simulink model "Model_InterpretationEngine64"  (R2022b)
settings: Solver=FixedStepDiscrete  StartTime=0.0  StopTime=5  RelTol=1e-3  EnableMultiTasking=on
InitFcn:
  | % Initialize model
  | ModelSettings=BTConfig.GetModelSettings();
  | 
  | ModelSettings.Validate();
  | 
  | ModelInit;
  | 
  | 
  | % load library data
  | GainLibrary_data;
  | % Load saved values from partition process
  | CapturedConstMask.LoadMapFromFile(bdroot)
  | % Load saved values from partition process
  | TSP_Mask.LoadMapFromFile(bdroot)
StartFcn:
  | % make sure all the simulated RTC requests are found
  | %RTC_SIM_OBJ.ValidateREQs();
undefined symbols (not defined in the file or in its folder): NumHFRefBPF, NumHFRefLPF
libraries: StateVar x112, TSP x56, FeaturePath x24
(part 2 of 5)

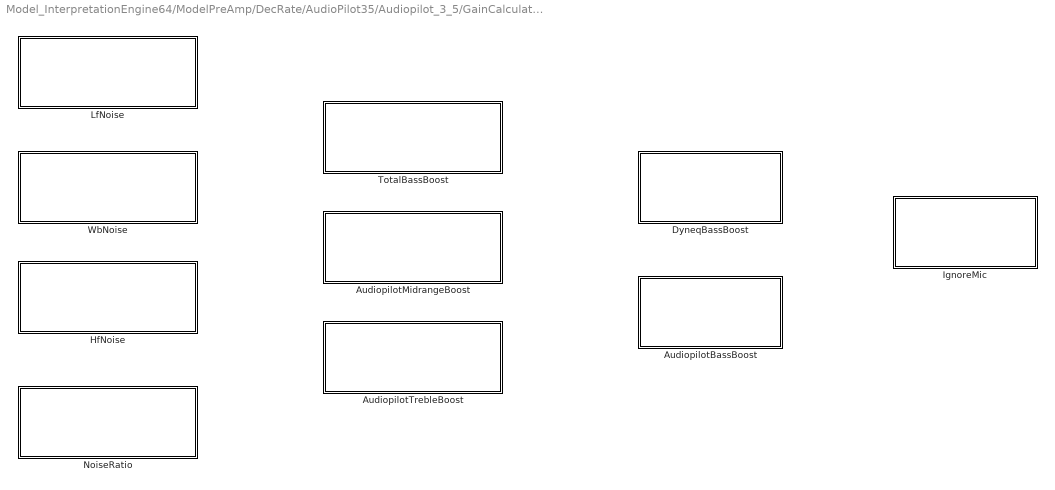
== system Model_InterpretationEngine64/ModelPreAmp/DecRate/AudioPilot35/Audiopilot_3_5/GainCalculation/Monitoring ==
  AudiopilotBassBoost : Subsystem  mask(Talaria Target State Variable){TriggerInit=[375 166 515 234], TspName=AudiopilotBassBoostDb, StateName=AudiopilotBassBoostDb, UseSameName=on, IfdefMacro=[]}
      mask prompts: TriggerInit "Hidden: MoveFcn redraw"; TspName "Name:"; StateName "Name of StateVar:"; UseSameName "Use same name for state variable and TSP"; IfdefMacro "Additional #ifdef macro to enable trigger capture:"
      mask help: The TargetStateVar block encapsultes a Target State Probe (TSP), a State Variable, and a Trivial Interpretation between them.
      mask init:
      | [ok,tspPath,activeStatePath] = TargetStateVarMask.Init(gcbh);
      settings: MoveFcn=TargetStateVarMask.CB_TriggerInit(gcbh);
      mask Help: See help for StateVar and TSP blocks
      mask Callback TriggerInit: TargetStateVarMask.CB_TriggerInit(gcbh);
      mask TypeOptions TspName: TSP/TspName
      mask TypeOptions StateName: StateVar/StateName
      mask Callback UseSameName: TargetStateVarMask.CB_UseSameName(gcbh);
      mask TypeOptions IfdefMacro: TSP/IfdefMacro
      mask DialogControl AdvancedPanel Prompt: Advanced
      mask DialogControl ConvertToFullInterpretation Prompt: Irreversible conversion to full interpretation
      mask DialogControl ConvertToFullInterpretation Callback: TargetStateVarMask.CB_ConvertToFullInterpretation(gcbh);
      mask DialogControl ErrorContainer Prompt: Error Messages
      mask DialogControl ErrorText Prompt: The interpreted StateVar value is not yet available
      mask DialogControl TspPathText Prompt: TSP: Current parameter name: [AudiopilotAudiopilotBassBoostDb]
      mask Display:
      | % retrieve icon definition
      | [path,w,h] = TargetStateVarMask.Icon();
      | 
      | % retrieve the block's pixel size
      | pos = get(gcbh,'position');
      | bw = pos(3) - pos(1);
      | bh = pos(4) - pos(2);
      | 
      | % draw centered icon
      | xAdj = bw/2 - w/2 + 5;
      | yAdj = bh/2 - h/2 + 4;
      | for i=1:length(path)
      | 	patch(path(i).x+xAdj, path(i).y+yAdj, path(i).rgb);
      | end
      | 
      | % show the top name or an X
      | if (exist('ok','var') && ok)
      | 	text(bw*0.5, bh*0.2, tspPath, 'horizontalAlignment', 'center');
      | 	patch(0,0,[1 1 1]);
      | 	patch(bw,bh,[1 1 1]);
      | else
      | 	tx=bw*0.03;
      | 	ty=bh*0.03;
      | 	patch([0 tx bw bw-tx], [ty 0 bh-ty bh], [1 0 0]);
      | 	patch([0 bw-tx bw tx], [bh-ty 0 ty bh], [1 0 0]);
      | end
  AudiopilotMidrangeBoost : Subsystem  mask(Talaria Target State Variable){TriggerInit=[60 101 235 169], TspName=AudiopilotMidrangeBoostDb, StateName=AudiopilotMidrangeBoostDb, UseSameName=on, IfdefMacro=[]}
      mask prompts: TriggerInit "Hidden: MoveFcn redraw"; TspName "Name:"; StateName "Name of StateVar:"; UseSameName "Use same name for state variable and TSP"; IfdefMacro "Additional #ifdef macro to enable trigger capture:"
      mask help: The TargetStateVar block encapsultes a Target State Probe (TSP), a State Variable, and a Trivial Interpretation between them.
      mask init:
      | [ok,tspPath,activeStatePath] = TargetStateVarMask.Init(gcbh);
      settings: MoveFcn=TargetStateVarMask.CB_TriggerInit(gcbh);
      mask Help: See help for StateVar and TSP blocks
      mask Callback TriggerInit: TargetStateVarMask.CB_TriggerInit(gcbh);
      mask TypeOptions TspName: TSP/TspName
      mask TypeOptions StateName: StateVar/StateName
      mask Callback UseSameName: TargetStateVarMask.CB_UseSameName(gcbh);
      mask TypeOptions IfdefMacro: TSP/IfdefMacro
      mask DialogControl AdvancedPanel Prompt: Advanced
      mask DialogControl ConvertToFullInterpretation Prompt: Irreversible conversion to full interpretation
      mask DialogControl ConvertToFullInterpretation Callback: TargetStateVarMask.CB_ConvertToFullInterpretation(gcbh);
      mask DialogControl ErrorContainer Prompt: Error Messages
      mask DialogControl ErrorText Prompt: The interpreted StateVar value is not yet available
      mask DialogControl TspPathText Prompt: TSP: Current parameter name: [AudiopilotAudiopilotMidrangeBoostDb]
      mask Display:
      | % retrieve icon definition
      | [path,w,h] = TargetStateVarMask.Icon();
      | 
      | % retrieve the block's pixel size
      | pos = get(gcbh,'position');
      | bw = pos(3) - pos(1);
      | bh = pos(4) - pos(2);
      | 
      | % draw centered icon
      | xAdj = bw/2 - w/2 + 5;
      | yAdj = bh/2 - h/2 + 4;
      | for i=1:length(path)
      | 	patch(path(i).x+xAdj, path(i).y+yAdj, path(i).rgb);
      | end
      | 
      | % show the top name or an X
      | if (exist('ok','var') && ok)
      | 	text(bw*0.5, bh*0.2, tspPath, 'horizontalAlignment', 'center');
      | 	patch(0,0,[1 1 1]);
      | 	patch(bw,bh,[1 1 1]);
      | else
      | 	tx=bw*0.03;
      | 	ty=bh*0.03;
      | 	patch([0 tx bw bw-tx], [ty 0 bh-ty bh], [1 0 0]);
      | 	patch([0 bw-tx bw tx], [bh-ty 0 ty bh], [1 0 0]);
      | end
  AudiopilotTrebleBoost : Subsystem  mask(Talaria Target State Variable){TriggerInit=[60 211 235 279], TspName=AudiopilotTrebleBoostDb, StateName=AudiopilotTrebleBoostDb, UseSameName=on, IfdefMacro=[]}
      mask prompts: TriggerInit "Hidden: MoveFcn redraw"; TspName "Name:"; StateName "Name of StateVar:"; UseSameName "Use same name for state variable and TSP"; IfdefMacro "Additional #ifdef macro to enable trigger capture:"
      mask help: The TargetStateVar block encapsultes a Target State Probe (TSP), a State Variable, and a Trivial Interpretation between them.
      mask init:
      | [ok,tspPath,activeStatePath] = TargetStateVarMask.Init(gcbh);
      settings: MoveFcn=TargetStateVarMask.CB_TriggerInit(gcbh);
      mask Help: See help for StateVar and TSP blocks
      mask Callback TriggerInit: TargetStateVarMask.CB_TriggerInit(gcbh);
      mask TypeOptions TspName: TSP/TspName
      mask TypeOptions StateName: StateVar/StateName
      mask Callback UseSameName: TargetStateVarMask.CB_UseSameName(gcbh);
      mask TypeOptions IfdefMacro: TSP/IfdefMacro
      mask DialogControl AdvancedPanel Prompt: Advanced
      mask DialogControl ConvertToFullInterpretation Prompt: Irreversible conversion to full interpretation
      mask DialogControl ConvertToFullInterpretation Callback: TargetStateVarMask.CB_ConvertToFullInterpretation(gcbh);
      mask DialogControl ErrorContainer Prompt: Error Messages
      mask DialogControl ErrorText Prompt: The interpreted StateVar value is not yet available
      mask DialogControl TspPathText Prompt: TSP: Current parameter name: [AudiopilotAudiopilotTrebleBoostDb]
      mask Display:
      | % retrieve icon definition
      | [path,w,h] = TargetStateVarMask.Icon();
      | 
      | % retrieve the block's pixel size
      | pos = get(gcbh,'position');
      | bw = pos(3) - pos(1);
      | bh = pos(4) - pos(2);
      | 
      | % draw centered icon
      | xAdj = bw/2 - w/2 + 5;
      | yAdj = bh/2 - h/2 + 4;
      | for i=1:length(path)
      | 	patch(path(i).x+xAdj, path(i).y+yAdj, path(i).rgb);
      | end
      | 
      | % show the top name or an X
      | if (exist('ok','var') && ok)
      | 	text(bw*0.5, bh*0.2, tspPath, 'horizontalAlignment', 'center');
      | 	patch(0,0,[1 1 1]);
      | 	patch(bw,bh,[1 1 1]);
      | else
      | 	tx=bw*0.03;
      | 	ty=bh*0.03;
      | 	patch([0 tx bw bw-tx], [ty 0 bh-ty bh], [1 0 0]);
      | 	patch([0 bw-tx bw tx], [bh-ty 0 ty bh], [1 0 0]);
      | end
  DyneqBassBoost : Subsystem  mask(Talaria Target State Variable){TriggerInit=[375 41 515 109], TspName=DyneqBassBoostDb, StateName=DyneqBassBoostDb, UseSameName=on, IfdefMacro=[]}
      mask prompts: TriggerInit "Hidden: MoveFcn redraw"; TspName "Name:"; StateName "Name of StateVar:"; UseSameName "Use same name for state variable and TSP"; IfdefMacro "Additional #ifdef macro to enable trigger capture:"
      mask help: The TargetStateVar block encapsultes a Target State Probe (TSP), a State Variable, and a Trivial Interpretation between them.
      mask init:
      | [ok,tspPath,activeStatePath] = TargetStateVarMask.Init(gcbh);
      settings: MoveFcn=TargetStateVarMask.CB_TriggerInit(gcbh);
      mask Help: See help for StateVar and TSP blocks
      mask Callback TriggerInit: TargetStateVarMask.CB_TriggerInit(gcbh);
      mask TypeOptions TspName: TSP/TspName
      mask TypeOptions StateName: StateVar/StateName
      mask Callback UseSameName: TargetStateVarMask.CB_UseSameName(gcbh);
      mask TypeOptions IfdefMacro: TSP/IfdefMacro
      mask DialogControl AdvancedPanel Prompt: Advanced
      mask DialogControl ConvertToFullInterpretation Prompt: Irreversible conversion to full interpretation
      mask DialogControl ConvertToFullInterpretation Callback: TargetStateVarMask.CB_ConvertToFullInterpretation(gcbh);
      mask DialogControl ErrorContainer Prompt: Error Messages
      mask DialogControl ErrorText Prompt: The interpreted StateVar value is not yet available
      mask DialogControl TspPathText Prompt: TSP: Current parameter name: [AudiopilotDyneqBassBoostDb]
      mask Display:
      | % retrieve icon definition
      | [path,w,h] = TargetStateVarMask.Icon();
      | 
      | % retrieve the block's pixel size
      | pos = get(gcbh,'position');
      | bw = pos(3) - pos(1);
      | bh = pos(4) - pos(2);
      | 
      | % draw centered icon
      | xAdj = bw/2 - w/2 + 5;
      | yAdj = bh/2 - h/2 + 4;
      | for i=1:length(path)
      | 	patch(path(i).x+xAdj, path(i).y+yAdj, path(i).rgb);
      | end
      | 
      | % show the top name or an X
      | if (exist('ok','var') && ok)
      | 	text(bw*0.5, bh*0.2, tspPath, 'horizontalAlignment', 'center');
      | 	patch(0,0,[1 1 1]);
      | 	patch(bw,bh,[1 1 1]);
      | else
      | 	tx=bw*0.03;
      | 	ty=bh*0.03;
      | 	patch([0 tx bw bw-tx], [ty 0 bh-ty bh], [1 0 0]);
      | 	patch([0 bw-tx bw tx], [bh-ty 0 ty bh], [1 0 0]);
      | end
  HfNoise : Subsystem  mask(Talaria Target State Variable){TriggerInit=[-245 151 -70 219], TspName=HfNoiseDbspl, StateName=HfNoiseDbspl, UseSameName=on, IfdefMacro=[]}
      mask prompts: TriggerInit "Hidden: MoveFcn redraw"; TspName "Name:"; StateName "Name of StateVar:"; UseSameName "Use same name for state variable and TSP"; IfdefMacro "Additional #ifdef macro to enable trigger capture:"
      mask help: The TargetStateVar block encapsultes a Target State Probe (TSP), a State Variable, and a Trivial Interpretation between them.
      mask init:
      | [ok,tspPath,activeStatePath] = TargetStateVarMask.Init(gcbh);
      settings: MoveFcn=TargetStateVarMask.CB_TriggerInit(gcbh);
      mask Help: See help for StateVar and TSP blocks
      mask Callback TriggerInit: TargetStateVarMask.CB_TriggerInit(gcbh);
      mask TypeOptions TspName: TSP/TspName
      mask TypeOptions StateName: StateVar/StateName
      mask Callback UseSameName: TargetStateVarMask.CB_UseSameName(gcbh);
      mask TypeOptions IfdefMacro: TSP/IfdefMacro
      mask DialogControl AdvancedPanel Prompt: Advanced
      mask DialogControl ConvertToFullInterpretation Prompt: Irreversible conversion to full interpretation
      mask DialogControl ConvertToFullInterpretation Callback: TargetStateVarMask.CB_ConvertToFullInterpretation(gcbh);
      mask DialogControl ErrorContainer Prompt: Error Messages
      mask DialogControl ErrorText Prompt: The interpreted StateVar value is not yet available
      mask DialogControl TspPathText Prompt: TSP: Current parameter name: [AudiopilotHfNoiseDbspl]
      mask Display:
      | % retrieve icon definition
      | [path,w,h] = TargetStateVarMask.Icon();
      | 
      | % retrieve the block's pixel size
      | pos = get(gcbh,'position');
      | bw = pos(3) - pos(1);
      | bh = pos(4) - pos(2);
      | 
      | % draw centered icon
      | xAdj = bw/2 - w/2 + 5;
      | yAdj = bh/2 - h/2 + 4;
      | for i=1:length(path)
      | 	patch(path(i).x+xAdj, path(i).y+yAdj, path(i).rgb);
      | end
      | 
      | % show the top name or an X
      | if (exist('ok','var') && ok)
      | 	text(bw*0.5, bh*0.2, tspPath, 'horizontalAlignment', 'center');
      | 	patch(0,0,[1 1 1]);
      | 	patch(bw,bh,[1 1 1]);
      | else
      | 	tx=bw*0.03;
      | 	ty=bh*0.03;
      | 	patch([0 tx bw bw-tx], [ty 0 bh-ty bh], [1 0 0]);
      | 	patch([0 bw-tx bw tx], [bh-ty 0 ty bh], [1 0 0]);
      | end
  IgnoreMic : Subsystem  mask(Talaria Target State Variable){TriggerInit=[630 86 770 154], TspName=IgnoreMicFlag, StateName=IgnoreMicFlag, UseSameName=on, IfdefMacro=[]}
      mask prompts: TriggerInit "Hidden: MoveFcn redraw"; TspName "Name:"; StateName "Name of StateVar:"; UseSameName "Use same name for state variable and TSP"; IfdefMacro "Additional #ifdef macro to enable trigger capture:"
      mask help: The TargetStateVar block encapsultes a Target State Probe (TSP), a State Variable, and a Trivial Interpretation between them.
      mask init:
      | [ok,tspPath,activeStatePath] = TargetStateVarMask.Init(gcbh);
      settings: MoveFcn=TargetStateVarMask.CB_TriggerInit(gcbh);
      mask Help: See help for StateVar and TSP blocks
      mask Callback TriggerInit: TargetStateVarMask.CB_TriggerInit(gcbh);
      mask TypeOptions TspName: TSP/TspName
      mask TypeOptions StateName: StateVar/StateName
      mask Callback UseSameName: TargetStateVarMask.CB_UseSameName(gcbh);
      mask TypeOptions IfdefMacro: TSP/IfdefMacro
      mask DialogControl AdvancedPanel Prompt: Advanced
      mask DialogControl ConvertToFullInterpretation Prompt: Irreversible conversion to full interpretation
      mask DialogControl ConvertToFullInterpretation Callback: TargetStateVarMask.CB_ConvertToFullInterpretation(gcbh);
      mask DialogControl ErrorContainer Prompt: Error Messages
      mask DialogControl ErrorText Prompt: The interpreted StateVar value is not yet available
      mask DialogControl TspPathText Prompt: TSP: Current parameter name: [AudiopilotIgnoreMicFlag]
      mask Display:
      | % retrieve icon definition
      | [path,w,h] = TargetStateVarMask.Icon();
      | 
      | % retrieve the block's pixel size
      | pos = get(gcbh,'position');
      | bw = pos(3) - pos(1);
      | bh = pos(4) - pos(2);
      | 
      | % draw centered icon
      | xAdj = bw/2 - w/2 + 5;
      | yAdj = bh/2 - h/2 + 4;
      | for i=1:length(path)
      | 	patch(path(i).x+xAdj, path(i).y+yAdj, path(i).rgb);
      | end
      | 
      | % show the top name or an X
      | if (exist('ok','var') && ok)
      | 	text(bw*0.5, bh*0.2, tspPath, 'horizontalAlignment', 'center');
      | 	patch(0,0,[1 1 1]);
      | 	patch(bw,bh,[1 1 1]);
      | else
      | 	tx=bw*0.03;
      | 	ty=bh*0.03;
      | 	patch([0 tx bw bw-tx], [ty 0 bh-ty bh], [1 0 0]);
      | 	patch([0 bw-tx bw tx], [bh-ty 0 ty bh], [1 0 0]);
      | end
  LfNoise : Subsystem  mask(Talaria Target State Variable){TriggerInit=[-245 -74 -70 -6], TspName=LfNoiseDbspl, StateName=LfNoiseDbspl, UseSameName=on, IfdefMacro=[]}
      mask prompts: TriggerInit "Hidden: MoveFcn redraw"; TspName "Name:"; StateName "Name of StateVar:"; UseSameName "Use same name for state variable and TSP"; IfdefMacro "Additional #ifdef macro to enable trigger capture:"
      mask help: The TargetStateVar block encapsultes a Target State Probe (TSP), a State Variable, and a Trivial Interpretation between them.
      mask init:
      | [ok,tspPath,activeStatePath] = TargetStateVarMask.Init(gcbh);
      settings: MoveFcn=TargetStateVarMask.CB_TriggerInit(gcbh);
      mask Help: See help for StateVar and TSP blocks
      mask Callback TriggerInit: TargetStateVarMask.CB_TriggerInit(gcbh);
      mask TypeOptions TspName: TSP/TspName
      mask TypeOptions StateName: StateVar/StateName
      mask Callback UseSameName: TargetStateVarMask.CB_UseSameName(gcbh);
      mask TypeOptions IfdefMacro: TSP/IfdefMacro
      mask DialogControl AdvancedPanel Prompt: Advanced
      mask DialogControl ConvertToFullInterpretation Prompt: Irreversible conversion to full interpretation
      mask DialogControl ConvertToFullInterpretation Callback: TargetStateVarMask.CB_ConvertToFullInterpretation(gcbh);
      mask DialogControl ErrorContainer Prompt: Error Messages
      mask DialogControl ErrorText Prompt: The interpreted StateVar value is not yet available
      mask DialogControl TspPathText Prompt: TSP: Current parameter name: [AudiopilotLfNoiseDbspl]
      mask Display:
      | % retrieve icon definition
      | [path,w,h] = TargetStateVarMask.Icon();
      | 
      | % retrieve the block's pixel size
      | pos = get(gcbh,'position');
      | bw = pos(3) - pos(1);
      | bh = pos(4) - pos(2);
      | 
      | % draw centered icon
      | xAdj = bw/2 - w/2 + 5;
      | yAdj = bh/2 - h/2 + 4;
      | for i=1:length(path)
      | 	patch(path(i).x+xAdj, path(i).y+yAdj, path(i).rgb);
      | end
      | 
      | % show the top name or an X
      | if (exist('ok','var') && ok)
      | 	text(bw*0.5, bh*0.2, tspPath, 'horizontalAlignment', 'center');
      | 	patch(0,0,[1 1 1]);
      | 	patch(bw,bh,[1 1 1]);
      | else
      | 	tx=bw*0.03;
      | 	ty=bh*0.03;
      | 	patch([0 tx bw bw-tx], [ty 0 bh-ty bh], [1 0 0]);
      | 	patch([0 bw-tx bw tx], [bh-ty 0 ty bh], [1 0 0]);
      | end
  NoiseRatio : Subsystem  mask(Talaria Target State Variable){TriggerInit=[-245 276 -70 344], TspName=NoiseRatio, StateName=NoiseRatio, UseSameName=on, IfdefMacro=[]}
      mask prompts: TriggerInit "Hidden: MoveFcn redraw"; TspName "Name:"; StateName "Name of StateVar:"; UseSameName "Use same name for state variable and TSP"; IfdefMacro "Additional #ifdef macro to enable trigger capture:"
      mask help: The TargetStateVar block encapsultes a Target State Probe (TSP), a State Variable, and a Trivial Interpretation between them.
      mask init:
      | [ok,tspPath,activeStatePath] = TargetStateVarMask.Init(gcbh);
      settings: MoveFcn=TargetStateVarMask.CB_TriggerInit(gcbh);
      mask Help: See help for StateVar and TSP blocks
      mask Callback TriggerInit: TargetStateVarMask.CB_TriggerInit(gcbh);
      mask TypeOptions TspName: TSP/TspName
      mask TypeOptions StateName: StateVar/StateName
      mask Callback UseSameName: TargetStateVarMask.CB_UseSameName(gcbh);
      mask TypeOptions IfdefMacro: TSP/IfdefMacro
      mask DialogControl AdvancedPanel Prompt: Advanced
      mask DialogControl ConvertToFullInterpretation Prompt: Irreversible conversion to full interpretation
      mask DialogControl ConvertToFullInterpretation Callback: TargetStateVarMask.CB_ConvertToFullInterpretation(gcbh);
      mask DialogControl ErrorContainer Prompt: Error Messages
      mask DialogControl ErrorText Prompt: The interpreted StateVar value is not yet available
      mask DialogControl TspPathText Prompt: TSP: Current parameter name: [AudiopilotNoiseRatio]
      mask Display:
      | % retrieve icon definition
      | [path,w,h] = TargetStateVarMask.Icon();
      | 
      | % retrieve the block's pixel size
      | pos = get(gcbh,'position');
      | bw = pos(3) - pos(1);
      | bh = pos(4) - pos(2);
      | 
      | % draw centered icon
      | xAdj = bw/2 - w/2 + 5;
      | yAdj = bh/2 - h/2 + 4;
      | for i=1:length(path)
      | 	patch(path(i).x+xAdj, path(i).y+yAdj, path(i).rgb);
      | end
      | 
      | % show the top name or an X
      | if (exist('ok','var') && ok)
      | 	text(bw*0.5, bh*0.2, tspPath, 'horizontalAlignment', 'center');
      | 	patch(0,0,[1 1 1]);
      | 	patch(bw,bh,[1 1 1]);
      | else
      | 	tx=bw*0.03;
      | 	ty=bh*0.03;
      | 	patch([0 tx bw bw-tx], [ty 0 bh-ty bh], [1 0 0]);
      | 	patch([0 bw-tx bw tx], [bh-ty 0 ty bh], [1 0 0]);
      | end
  TotalBassBoost : Subsystem  mask(Talaria Target State Variable){TriggerInit=[60 -9 235 59], TspName=TotalBassBoostDb, StateName=TotalBassBoostDb, UseSameName=on, IfdefMacro=[]}
      mask prompts: TriggerInit "Hidden: MoveFcn redraw"; TspName "Name:"; StateName "Name of StateVar:"; UseSameName "Use same name for state variable and TSP"; IfdefMacro "Additional #ifdef macro to enable trigger capture:"
      mask help: The TargetStateVar block encapsultes a Target State Probe (TSP), a State Variable, and a Trivial Interpretation between them.
      mask init:
      | [ok,tspPath,activeStatePath] = TargetStateVarMask.Init(gcbh);
      settings: MoveFcn=TargetStateVarMask.CB_TriggerInit(gcbh);
      mask Help: See help for StateVar and TSP blocks
      mask Callback TriggerInit: TargetStateVarMask.CB_TriggerInit(gcbh);
      mask TypeOptions TspName: TSP/TspName
      mask TypeOptions StateName: StateVar/StateName
      mask Callback UseSameName: TargetStateVarMask.CB_UseSameName(gcbh);
      mask TypeOptions IfdefMacro: TSP/IfdefMacro
      mask DialogControl AdvancedPanel Prompt: Advanced
      mask DialogControl ConvertToFullInterpretation Prompt: Irreversible conversion to full interpretation
      mask DialogControl ConvertToFullInterpretation Callback: TargetStateVarMask.CB_ConvertToFullInterpretation(gcbh);
      mask DialogControl ErrorContainer Prompt: Error Messages
      mask DialogControl ErrorText Prompt: The interpreted StateVar value is not yet available
      mask DialogControl TspPathText Prompt: TSP: Current parameter name: [AudiopilotTotalBassBoostDb]
      mask Display:
      | % retrieve icon definition
      | [path,w,h] = TargetStateVarMask.Icon();
      | 
      | % retrieve the block's pixel size
      | pos = get(gcbh,'position');
      | bw = pos(3) - pos(1);
      | bh = pos(4) - pos(2);
      | 
      | % draw centered icon
      | xAdj = bw/2 - w/2 + 5;
      | yAdj = bh/2 - h/2 + 4;
      | for i=1:length(path)
      | 	patch(path(i).x+xAdj, path(i).y+yAdj, path(i).rgb);
      | end
      | 
      | % show the top name or an X
      | if (exist('ok','var') && ok)
      | 	text(bw*0.5, bh*0.2, tspPath, 'horizontalAlignment', 'center');
      | 	patch(0,0,[1 1 1]);
      | 	patch(bw,bh,[1 1 1]);
      | else
      | 	tx=bw*0.03;
      | 	ty=bh*0.03;
      | 	patch([0 tx bw bw-tx], [ty 0 bh-ty bh], [1 0 0]);
      | 	patch([0 bw-tx bw tx], [bh-ty 0 ty bh], [1 0 0]);
      | end
  WbNoise : Subsystem  mask(Talaria Target State Variable){TriggerInit=[-245 41 -70 109], TspName=WbNoiseDbspl, StateName=WbNoiseDbspl, UseSameName=on, IfdefMacro=[]}
      mask prompts: TriggerInit "Hidden: MoveFcn redraw"; TspName "Name:"; StateName "Name of StateVar:"; UseSameName "Use same name for state variable and TSP"; IfdefMacro "Additional #ifdef macro to enable trigger capture:"
      mask help: The TargetStateVar block encapsultes a Target State Probe (TSP), a State Variable, and a Trivial Interpretation between them.
      mask init:
      | [ok,tspPath,activeStatePath] = TargetStateVarMask.Init(gcbh);
      settings: MoveFcn=TargetStateVarMask.CB_TriggerInit(gcbh);
      mask Help: See help for StateVar and TSP blocks
      mask Callback TriggerInit: TargetStateVarMask.CB_TriggerInit(gcbh);
      mask TypeOptions TspName: TSP/TspName
      mask TypeOptions StateName: StateVar/StateName
      mask Callback UseSameName: TargetStateVarMask.CB_UseSameName(gcbh);
      mask TypeOptions IfdefMacro: TSP/IfdefMacro
      mask DialogControl AdvancedPanel Prompt: Advanced
      mask DialogControl ConvertToFullInterpretation Prompt: Irreversible conversion to full interpretation
      mask DialogControl ConvertToFullInterpretation Callback: TargetStateVarMask.CB_ConvertToFullInterpretation(gcbh);
      mask DialogControl ErrorContainer Prompt: Error Messages
      mask DialogControl ErrorText Prompt: The interpreted StateVar value is not yet available
      mask DialogControl TspPathText Prompt: TSP: Current parameter name: [AudiopilotWbNoiseDbspl]
      mask Display:
      | % retrieve icon definition
      | [path,w,h] = TargetStateVarMask.Icon();
      | 
      | % retrieve the block's pixel size
      | pos = get(gcbh,'position');
      | bw = pos(3) - pos(1);
      | bh = pos(4) - pos(2);
      | 
      | % draw centered icon
      | xAdj = bw/2 - w/2 + 5;
      | yAdj = bh/2 - h/2 + 4;
      | for i=1:length(path)
      | 	patch(path(i).x+xAdj, path(i).y+yAdj, path(i).rgb);
      | end
      | 
      | % show the top name or an X
      | if (exist('ok','var') && ok)
      | 	text(bw*0.5, bh*0.2, tspPath, 'horizontalAlignment', 'center');
      | 	patch(0,0,[1 1 1]);
      | 	patch(bw,bh,[1 1 1]);
      | else
      | 	tx=bw*0.03;
      | 	ty=bh*0.03;
      | 	patch([0 tx bw bw-tx], [ty 0 bh-ty bh], [1 0 0]);
      | 	patch([0 bw-tx bw tx], [bh-ty 0 ty bh], [1 0 0]);
      | end

== system Model_InterpretationEngine64/ModelPreAmp/DecRate/AudioPilot35/Audiopilot_3_5/GainCalculation/RampedEnable ==
  audiopilot boost gain : Subsystem  mask(Talaria Target State Variable){TriggerInit=[185 -359 325 -291], TspName=AudiopilotBoostGain, StateName=AudiopilotBoostGain, UseSameName=on, IfdefMacro=[]}
      mask prompts: TriggerInit "Hidden: MoveFcn redraw"; TspName "Name:"; StateName "Name of StateVar:"; UseSameName "Use same name for state variable and TSP"; IfdefMacro "Additional #ifdef macro to enable trigger capture:"
      mask help: The TargetStateVar block encapsultes a Target State Probe (TSP), a State Variable, and a Trivial Interpretation between them.
      mask init:
      | [ok,tspPath,activeStatePath] = TargetStateVarMask.Init(gcbh);
      settings: MoveFcn=TargetStateVarMask.CB_TriggerInit(gcbh);
      mask Help: See help for StateVar and TSP blocks
      mask Callback TriggerInit: TargetStateVarMask.CB_TriggerInit(gcbh);
      mask TypeOptions TspName: TSP/TspName
      mask TypeOptions StateName: StateVar/StateName
      mask Callback UseSameName: TargetStateVarMask.CB_UseSameName(gcbh);
      mask TypeOptions IfdefMacro: TSP/IfdefMacro
      mask DialogControl AdvancedPanel Prompt: Advanced
      mask DialogControl ConvertToFullInterpretation Prompt: Irreversible conversion to full interpretation
      mask DialogControl ConvertToFullInterpretation Callback: TargetStateVarMask.CB_ConvertToFullInterpretation(gcbh);
      mask DialogControl ErrorContainer Prompt: Error Messages
      mask DialogControl ErrorText Prompt: The interpreted StateVar value is not yet available
      mask DialogControl TspPathText Prompt: TSP: Current parameter name: [AudiopilotAudiopilotBoostGain]
      mask Display:
      | % retrieve icon definition
      | [path,w,h] = TargetStateVarMask.Icon();
      | 
      | % retrieve the block's pixel size
      | pos = get(gcbh,'position');
      | bw = pos(3) - pos(1);
      | bh = pos(4) - pos(2);
      | 
      | % draw centered icon
      | xAdj = bw/2 - w/2 + 5;
      | yAdj = bh/2 - h/2 + 4;
      | for i=1:length(path)
      | 	patch(path(i).x+xAdj, path(i).y+yAdj, path(i).rgb);
      | end
      | 
      | % show the top name or an X
      | if (exist('ok','var') && ok)
      | 	text(bw*0.5, bh*0.2, tspPath, 'horizontalAlignment', 'center');
      | 	patch(0,0,[1 1 1]);
      | 	patch(bw,bh,[1 1 1]);
      | else
      | 	tx=bw*0.03;
      | 	ty=bh*0.03;
      | 	patch([0 tx bw bw-tx], [ty 0 bh-ty bh], [1 0 0]);
      | 	patch([0 bw-tx bw tx], [bh-ty 0 ty bh], [1 0 0]);
      | end
  dyneq boost gain : Subsystem  mask(Talaria Target State Variable){TriggerInit=[185 -454 325 -386], TspName=DyneqBoostGain, StateName=DyneqBoostGain, UseSameName=on, IfdefMacro=[]}
      mask prompts: TriggerInit "Hidden: MoveFcn redraw"; TspName "Name:"; StateName "Name of StateVar:"; UseSameName "Use same name for state variable and TSP"; IfdefMacro "Additional #ifdef macro to enable trigger capture:"
      mask help: The TargetStateVar block encapsultes a Target State Probe (TSP), a State Variable, and a Trivial Interpretation between them.
      mask init:
      | [ok,tspPath,activeStatePath] = TargetStateVarMask.Init(gcbh);
      settings: MoveFcn=TargetStateVarMask.CB_TriggerInit(gcbh);
      mask Help: See help for StateVar and TSP blocks
      mask Callback TriggerInit: TargetStateVarMask.CB_TriggerInit(gcbh);
      mask TypeOptions TspName: TSP/TspName
      mask TypeOptions StateName: StateVar/StateName
      mask Callback UseSameName: TargetStateVarMask.CB_UseSameName(gcbh);
      mask TypeOptions IfdefMacro: TSP/IfdefMacro
      mask DialogControl AdvancedPanel Prompt: Advanced
      mask DialogControl ConvertToFullInterpretation Prompt: Irreversible conversion to full interpretation
      mask DialogControl ConvertToFullInterpretation Callback: TargetStateVarMask.CB_ConvertToFullInterpretation(gcbh);
      mask DialogControl ErrorContainer Prompt: Error Messages
      mask DialogControl ErrorText Prompt: The interpreted StateVar value is not yet available
      mask DialogControl TspPathText Prompt: TSP: Current parameter name: [AudiopilotDyneqBoostGain]
      mask Display:
      | % retrieve icon definition
      | [path,w,h] = TargetStateVarMask.Icon();
      | 
      | % retrieve the block's pixel size
      | pos = get(gcbh,'position');
      | bw = pos(3) - pos(1);
      | bh = pos(4) - pos(2);
      | 
      | % draw centered icon
      | xAdj = bw/2 - w/2 + 5;
      | yAdj = bh/2 - h/2 + 4;
      | for i=1:length(path)
      | 	patch(path(i).x+xAdj, path(i).y+yAdj, path(i).rgb);
      | end
      | 
      | % show the top name or an X
      | if (exist('ok','var') && ok)
      | 	text(bw*0.5, bh*0.2, tspPath, 'horizontalAlignment', 'center');
      | 	patch(0,0,[1 1 1]);
      | 	patch(bw,bh,[1 1 1]);
      | else
      | 	tx=bw*0.03;
      | 	ty=bh*0.03;
      | 	patch([0 tx bw bw-tx], [ty 0 bh-ty bh], [1 0 0]);
      | 	patch([0 bw-tx bw tx], [bh-ty 0 ty bh], [1 0 0]);
      | end

== system Model_InterpretationEngine64/ModelPreAmp/DecRate/AudioPilot35/Audiopilot_3_5/NoiseEstimationVariant/RegularNoiseEstimation ==
  HFNoiseEstimatorCoh : Subsystem  mask(AudioPilot - High-Frequency Noise Estimator){FeatureName=HfNoise, NumHFRefLPF=NumHFRefLPF, NumHFRefBPF=NumHFRefBPF, Config=Config.HfNoise, TriggerInit=0}
      mask prompts: FeatureName "Feature Name:"; NumHFRefLPF "Number of "High-Pass" Reference Channels"; NumHFRefBPF "Number of "Full-Band" Reference Channels"; Config "HighFrequencyNoiseEstimatorCohConfig"
      mask help: This block implements the high-frequency noise estimator based on the multi-coherence method.
      mask init:
      | blkh = gcbh;
      | 
      | Config = BTConfig.Assert(blkh,Config);
      | Config.Validate();
      | 
      | % Matlab Function Parameters
      | FrameSize = Config.FrameSize;
      | SampleRate = Config.SampleRateHz;
      | HFDecRate = Config.DecRateHz;
      | HFDecRate2 = Config.CoherenceDecRateHz;
      | HFDecRate3 = Config.CoherenceDecRate2Hz;   
      | 
      | % Constants
      | 
      | EmptyStftInput = zeros((FrameSize/Config.DecimationFactor),1);
      |           
      | % Create the PoolIIR Coefficients and Parameters           
      | [AA, BPLP, NumAAChannels, NumHFRefChannels] ...
      |     = HighFrequencyNoiseEstimatorCohMask.FormFilterCoef ...
      |                 (blkh,Config,NumHFRefLPF,NumHFRefBPF);
      | 
      | % Configure Model according to Mask & Config Parameters            
      | HighFrequencyNoiseEstimatorCohMask.ConfigureModel ...
      |                 (blkh,NumHFRefLPF,NumHFRefBPF,Config);
      | 
      | BTConfig.InitSetFeatureIfPresent(blkh,'FeatureName');
      mask Help:
      | Arguments for this block:
      | 
      | Design Time Configuration
      | 
      | Feature Name -
      | The Feature Name can be specified unless a BTC instance is used, in which case, the instance name will be used as Feature Name.
      | 
      | Number of "High-Pass"Reference Channels -
      | These are the reference channels from Medusa that have already been high-passed, such as  Limp, Rimp etc.  These channels will then undergo low-pass filtering only.
      | 
      | Number of "Full-Band" Reference Channels -
      | These are the reference channels from Medusa that are essentially full-band, such as LStreb, RStreb etc.  These channels will then undergo band-pass filtering.
      | 
      | Build Time Configuration -
      | The block can be configured using a object of class, HighFrequencyNoiseEstimatorCohConfig.
      mask TypeOptions FeatureName: FeaturePath/FeatureName
      mask Callback Config: BTConfig.CallbackHideIfPresent(gcbh,{'FeatureName'});
      mask Callback TriggerInit: HighFrequencyNoiseEstimatorCohMask.TriggerInitCallBack(gcbh);
      mask DialogControl DTCTitle Prompt: <b>Design Time Configuration</b>
      mask DialogControl BTCTitle Prompt: <b>Build Time Configuration</b>
  LFNoiseEstimatorCoh : Subsystem  mask(AudioPilot - Low-Frequency Noise Estimator){FeatureName=LfNoise, Config=Config.LfNoise, TriggerInit=0}
      mask prompts: FeatureName "Feature Name:"; Config "LowFrequencyNoiseEstimatorCohConfig"
      mask help: This block implements the low-frequency noise estimator using the multi-coherence method.
      mask init:
      | blkh = gcbh;
      | 
      | Config = BTConfig.Assert(blkh,Config);
      | Config.Validate();
      | 
      | DecRate = Config.DecRateHz;
      | DecRate2 = Config.CoherenceDecRateHz;
      | DecRate3 = Config.CoherenceDecRate2Hz;
      | 
      | LowFrequencyNoiseEstimatorCohMask.ConfigureModel ...
      |                 (blkh,Config)
      | 
      | BTConfig.InitSetFeatureIfPresent(blkh,'FeatureName');
      mask Help:
      | This block implements the low-frequency noise estimator using the multi-coherence method.
      | 
      | Arguments for this block:
      | 
      | Design Time Configuration
      | The Feature Name can be specified unless a BTC instance is used, in which case, the instance name will be used as Feature Name.
      | 
      | Build Time Configuration
      | The block can be configured using a BTC object, LowFrequencyNoiseEstimatorCohConfig.
      mask TypeOptions FeatureName: FeaturePath/FeatureName
      mask Callback Config: BTConfig.CallbackHideIfPresent(gcbh,{'FeatureName'});
      mask Callback TriggerInit: LowFrequencyNoiseEstimatorCohMask.TriggerInitCallBack(gcbh);
      mask DialogControl DTCTitle Prompt: <b> Design Time Configuration </b>
      mask DialogControl BTCTitle Prompt: <b> Build Time Configuration </b>
      mask DialogControl Config Tooltip: The configuration has to be an object of the class, LowFrequencyNoiseEstimatorCohConfig.
  RatioCalculation : Subsystem  mask(AudioPilot - Noise Ratio Calculation){FeatureName=Ratio, Config=Config.Ratio}
      mask prompts: FeatureName "Feature Name:"; Config "RatioCalculationConfig"
      mask help: This block handles the computation, smoothing and impulse rejection of the noise ratio.
      mask init:
      | blkh = gcbh;
      | 
      | Config = BTConfig.Assert(blkh,Config);
      | Config.Validate();
      | 
      | SampleRate = Config.SampleRateHz;
      | HFDecRate = Config.DecRateHz;
      |  
      | BTConfig.InitSetFeatureIfPresent(blkh,'FeatureName');
      mask Help:
      | This block handles the computation, smoothing and impulse rejection of the noise ratio.
      | 
      | Arguments for this block:
      | 
      | Design Time Configuration
      | The Feature Name can be specified unless a BTC instance is used, in which case, the instance name will be used as Feature Name.
      | 
      | Build Time Configuration
      | The block can be configured using a object of class, RatioCalculationConfig.
      mask TypeOptions FeatureName: FeaturePath/FeatureName
      mask Callback Config: BTConfig.CallbackHideIfPresent(gcbh,{'FeatureName'});
      mask DialogControl DTCTitle Prompt: <b>Design Time Configuration </b>
      mask DialogControl BTCTitle Prompt: <b>Build Time Configuration </b>
      mask DialogControl Config Tooltip: The configuration has to be an object of the class, RatioCalculationConfig.

== system Model_InterpretationEngine64/ModelPreAmp/DecRate/AudioPilot35/Audiopilot_3_5/NoiseEstimationVariant/SpeedOnly ==

== system Model_InterpretationEngine64/ModelPreAmp/DecRate/AudioPilot35/EntertainmentLevelDetection/AudiopilotLevelDetect/Monitor ==
  FeaturePath : FeaturePath/FeaturePath  FeatureName=LevelWatchAudiopilot  IsGroup=off  GroupNumber=-1  IsModule=off  TriggerInit=[620 -136 735 -29]
      settings: SourceProductName=Bose Talaria
  env : Subsystem  mask(Talaria Target State Variable){TriggerInit=[620 16 815 84], TspName=EnvDb, StateName=EnvDb, UseSameName=on, IfdefMacro=[]}
      mask prompts: TriggerInit "Hidden: MoveFcn redraw"; TspName "Name:"; StateName "Name of StateVar:"; UseSameName "Use same name for state variable and TSP"; IfdefMacro "Additional #ifdef macro to enable trigger capture:"
      mask help: The TargetStateVar block encapsultes a Target State Probe (TSP), a State Variable, and a Trivial Interpretation between them.
      mask init:
      | [ok,tspPath,activeStatePath] = TargetStateVarMask.Init(gcbh);
      settings: MoveFcn=TargetStateVarMask.CB_TriggerInit(gcbh);
      mask Help: See help for StateVar and TSP blocks
      mask Callback TriggerInit: TargetStateVarMask.CB_TriggerInit(gcbh);
      mask TypeOptions TspName: TSP/TspName
      mask TypeOptions StateName: StateVar/StateName
      mask Callback UseSameName: TargetStateVarMask.CB_UseSameName(gcbh);
      mask TypeOptions IfdefMacro: TSP/IfdefMacro
      mask DialogControl AdvancedPanel Prompt: Advanced
      mask DialogControl ConvertToFullInterpretation Prompt: Irreversible conversion to full interpretation
      mask DialogControl ConvertToFullInterpretation Callback: TargetStateVarMask.CB_ConvertToFullInterpretation(gcbh);
      mask DialogControl ErrorContainer Prompt: Error Messages
      mask DialogControl ErrorText Prompt: The interpreted StateVar value is not yet available
      mask DialogControl TspPathText Prompt: TSP: Current parameter name: [PreAmpLevelWatchAudiopilotEnvDb]
      mask Display:
      | % retrieve icon definition
      | [path,w,h] = TargetStateVarMask.Icon();
      | 
      | % retrieve the block's pixel size
      | pos = get(gcbh,'position');
      | bw = pos(3) - pos(1);
      | bh = pos(4) - pos(2);
      | 
      | % draw centered icon
      | xAdj = bw/2 - w/2 + 5;
      | yAdj = bh/2 - h/2 + 4;
      | for i=1:length(path)
      | 	patch(path(i).x+xAdj, path(i).y+yAdj, path(i).rgb);
      | end
      | 
      | % show the top name or an X
      | if (exist('ok','var') && ok)
      | 	text(bw*0.5, bh*0.2, tspPath, 'horizontalAlignment', 'center');
      | 	patch(0,0,[1 1 1]);
      | 	patch(bw,bh,[1 1 1]);
      | else
      | 	tx=bw*0.03;
      | 	ty=bh*0.03;
      | 	patch([0 tx bw bw-tx], [ty 0 bh-ty bh], [1 0 0]);
      | 	patch([0 bw-tx bw tx], [bh-ty 0 ty bh], [1 0 0]);
      | end
  level : Subsystem  mask(Talaria Target State Variable){TriggerInit=[620 126 815 194], TspName=LevelDbspl, StateName=LevelDbspl, UseSameName=on, IfdefMacro=[]}
      mask prompts: TriggerInit "Hidden: MoveFcn redraw"; TspName "Name:"; StateName "Name of StateVar:"; UseSameName "Use same name for state variable and TSP"; IfdefMacro "Additional #ifdef macro to enable trigger capture:"
      mask help: The TargetStateVar block encapsultes a Target State Probe (TSP), a State Variable, and a Trivial Interpretation between them.
      mask init:
      | [ok,tspPath,activeStatePath] = TargetStateVarMask.Init(gcbh);
      settings: MoveFcn=TargetStateVarMask.CB_TriggerInit(gcbh);
      mask Help: See help for StateVar and TSP blocks
      mask Callback TriggerInit: TargetStateVarMask.CB_TriggerInit(gcbh);
      mask TypeOptions TspName: TSP/TspName
      mask TypeOptions StateName: StateVar/StateName
      mask Callback UseSameName: TargetStateVarMask.CB_UseSameName(gcbh);
      mask TypeOptions IfdefMacro: TSP/IfdefMacro
      mask DialogControl AdvancedPanel Prompt: Advanced
      mask DialogControl ConvertToFullInterpretation Prompt: Irreversible conversion to full interpretation
      mask DialogControl ConvertToFullInterpretation Callback: TargetStateVarMask.CB_ConvertToFullInterpretation(gcbh);
      mask DialogControl ErrorContainer Prompt: Error Messages
      mask DialogControl ErrorText Prompt: The interpreted StateVar value is not yet available
      mask DialogControl TspPathText Prompt: TSP: Current parameter name: [PreAmpLevelWatchAudiopilotLevelDbspl]
      mask Display:
      | % retrieve icon definition
      | [path,w,h] = TargetStateVarMask.Icon();
      | 
      | % retrieve the block's pixel size
      | pos = get(gcbh,'position');
      | bw = pos(3) - pos(1);
      | bh = pos(4) - pos(2);
      | 
      | % draw centered icon
      | xAdj = bw/2 - w/2 + 5;
      | yAdj = bh/2 - h/2 + 4;
      | for i=1:length(path)
      | 	patch(path(i).x+xAdj, path(i).y+yAdj, path(i).rgb);
      | end
      | 
      | % show the top name or an X
      | if (exist('ok','var') && ok)
      | 	text(bw*0.5, bh*0.2, tspPath, 'horizontalAlignment', 'center');
      | 	patch(0,0,[1 1 1]);
      | 	patch(bw,bh,[1 1 1]);
      | else
      | 	tx=bw*0.03;
      | 	ty=bh*0.03;
      | 	patch([0 tx bw bw-tx], [ty 0 bh-ty bh], [1 0 0]);
      | 	patch([0 bw-tx bw tx], [bh-ty 0 ty bh], [1 0 0]);
      | end

== system Model_InterpretationEngine64/ModelPreAmp/DecRate/AudioPilot35/EntertainmentLevelDetection/DyneqLevelDetect/Monitor ==
  FeaturePath : FeaturePath/FeaturePath  FeatureName=LevelWatchDyneq  IsGroup=off  GroupNumber=-1  IsModule=off  TriggerInit=[300 -156 415 -49]
      settings: SourceProductName=Bose Talaria
  env : Subsystem  mask(Talaria Target State Variable){TriggerInit=[300 16 495 84], TspName=EnvDb, StateName=EnvDb, UseSameName=on, IfdefMacro=[]}
      mask prompts: TriggerInit "Hidden: MoveFcn redraw"; TspName "Name:"; StateName "Name of StateVar:"; UseSameName "Use same name for state variable and TSP"; IfdefMacro "Additional #ifdef macro to enable trigger capture:"
      mask help: The TargetStateVar block encapsultes a Target State Probe (TSP), a State Variable, and a Trivial Interpretation between them.
      mask init:
      | [ok,tspPath,activeStatePath] = TargetStateVarMask.Init(gcbh);
      settings: MoveFcn=TargetStateVarMask.CB_TriggerInit(gcbh);
      mask Help: See help for StateVar and TSP blocks
      mask Callback TriggerInit: TargetStateVarMask.CB_TriggerInit(gcbh);
      mask TypeOptions TspName: TSP/TspName
      mask TypeOptions StateName: StateVar/StateName
      mask Callback UseSameName: TargetStateVarMask.CB_UseSameName(gcbh);
      mask TypeOptions IfdefMacro: TSP/IfdefMacro
      mask DialogControl AdvancedPanel Prompt: Advanced
      mask DialogControl ConvertToFullInterpretation Prompt: Irreversible conversion to full interpretation
      mask DialogControl ConvertToFullInterpretation Callback: TargetStateVarMask.CB_ConvertToFullInterpretation(gcbh);
      mask DialogControl ErrorContainer Prompt: Error Messages
      mask DialogControl ErrorText Prompt: The interpreted StateVar value is not yet available
      mask DialogControl TspPathText Prompt: TSP: Current parameter name: [PreAmpLevelWatchDyneqEnvDb]
      mask Display:
      | % retrieve icon definition
      | [path,w,h] = TargetStateVarMask.Icon();
      | 
      | % retrieve the block's pixel size
      | pos = get(gcbh,'position');
      | bw = pos(3) - pos(1);
      | bh = pos(4) - pos(2);
      | 
      | % draw centered icon
      | xAdj = bw/2 - w/2 + 5;
      | yAdj = bh/2 - h/2 + 4;
      | for i=1:length(path)
      | 	patch(path(i).x+xAdj, path(i).y+yAdj, path(i).rgb);
      | end
      | 
      | % show the top name or an X
      | if (exist('ok','var') && ok)
      | 	text(bw*0.5, bh*0.2, tspPath, 'horizontalAlignment', 'center');
      | 	patch(0,0,[1 1 1]);
      | 	patch(bw,bh,[1 1 1]);
      | else
      | 	tx=bw*0.03;
      | 	ty=bh*0.03;
      | 	patch([0 tx bw bw-tx], [ty 0 bh-ty bh], [1 0 0]);
      | 	patch([0 bw-tx bw tx], [bh-ty 0 ty bh], [1 0 0]);
      | end
  level : Subsystem  mask(Talaria Target State Variable){TriggerInit=[300 130 500 200], TspName=LevelDbspl, StateName=LevelDbspl, UseSameName=on, IfdefMacro=[]}
      mask prompts: TriggerInit "Hidden: MoveFcn redraw"; TspName "Name:"; StateName "Name of StateVar:"; UseSameName "Use same name for state variable and TSP"; IfdefMacro "Additional #ifdef macro to enable trigger capture:"
      mask help: The TargetStateVar block encapsultes a Target State Probe (TSP), a State Variable, and a Trivial Interpretation between them.
      mask init:
      | [ok,tspPath,activeStatePath] = TargetStateVarMask.Init(gcbh);
      settings: MoveFcn=TargetStateVarMask.CB_TriggerInit(gcbh);
      mask Help: See help for StateVar and TSP blocks
      mask Callback TriggerInit: TargetStateVarMask.CB_TriggerInit(gcbh);
      mask TypeOptions TspName: TSP/TspName
      mask TypeOptions StateName: StateVar/StateName
      mask Callback UseSameName: TargetStateVarMask.CB_UseSameName(gcbh);
      mask TypeOptions IfdefMacro: TSP/IfdefMacro
      mask DialogControl AdvancedPanel Prompt: Advanced
      mask DialogControl ConvertToFullInterpretation Prompt: Irreversible conversion to full interpretation
      mask DialogControl ConvertToFullInterpretation Callback: TargetStateVarMask.CB_ConvertToFullInterpretation(gcbh);
      mask DialogControl ErrorContainer Prompt: Error Messages
      mask DialogControl ErrorText Prompt: The interpreted StateVar value is not yet available
      mask DialogControl TspPathText Prompt: TSP: Current parameter name: [PreAmpLevelWatchDyneqLevelDbspl]
      mask Display:
      | % retrieve icon definition
      | [path,w,h] = TargetStateVarMask.Icon();
      | 
      | % retrieve the block's pixel size
      | pos = get(gcbh,'position');
      | bw = pos(3) - pos(1);
      | bh = pos(4) - pos(2);
      | 
      | % draw centered icon
      | xAdj = bw/2 - w/2 + 5;
      | yAdj = bh/2 - h/2 + 4;
      | for i=1:length(path)
      | 	patch(path(i).x+xAdj, path(i).y+yAdj, path(i).rgb);
      | end
      | 
      | % show the top name or an X
      | if (exist('ok','var') && ok)
      | 	text(bw*0.5, bh*0.2, tspPath, 'horizontalAlignment', 'center');
      | 	patch(0,0,[1 1 1]);
      | 	patch(bw,bh,[1 1 1]);
      | else
      | 	tx=bw*0.03;
      | 	ty=bh*0.03;
      | 	patch([0 tx bw bw-tx], [ty 0 bh-ty bh], [1 0 0]);
      | 	patch([0 bw-tx bw tx], [bh-ty 0 ty bh], [1 0 0]);
      | end

== system Model_InterpretationEngine64/ModelPreAmp/DecRate/Medusa5H1/MedusaHoligram/Medusa5H1 Part 1/CAE Treble Boost ==
  note: 1) Add Subsystem or Model blocks as valid variant choices.
      | 2) You cannot connect blocks at this level. At simulation, connectivity is automatically
      | determined, based on the active variant and port name matching.
  Audio Passthrough : Subsystem  VariantControl=sys_defs.include_compressed_audio_enhancement == 0
  CAE Treble Boost : Subsystem  VariantControl=sys_defs.include_compressed_audio_enhancement == 1
